simulink model "decoderapp"  (R2017b)
settings: Solver=FixedStepAuto  StartTime=0.0  StopTime=inf  RelTol=1e-3
libraries: androidlib x10, dspstat3 x2
settings Model: Creator=eslac_000  LastModifiedBy=eslac_000
settings OptimizationCC: PassReuseOutputArgsAs=Individual arguments  MaxStackSize=64
settings DebuggingCC: ParameterTunabilityLossMsg=error
settings HardwareCC: ProdBitPerPointer=32  ProdBitPerSizeT=32  ProdBitPerPtrDiffT=32  ProdLargestAtomicInteger=Long  ProdLargestAtomicFloat=Double  ProdWordSize=32  ProdHWDeviceType=ARM Compatible->ARM Cortex
settings SFSimCC: MATLABDynamicMemAlloc=off
settings RTWCC: SystemTargetFile=ert.tlc  HardwareBoard=Android Device  TemplateMakefile=ert_default_tmf  GenerateReport=on  Toolchain=Android SDK/NDK Tools  IncludeHyperlinkInReport=on  LaunchReport=on  GenerateTraceInfo=on  GenerateTraceReport=on  GenerateTraceReportSl=on  GenerateTraceReportSf=on  GenerateTraceReportEml=on
settings CodeAppCC: ForceParamTrailComments=on  IgnoreCustomStorageClasses=off  OperatorAnnotations=on  SimulinkDataObjDesc=on  SFDataObjDesc=on  InsertBlockDesc=on
settings ERTTargetCC: SupportVariableSizeSignals=on

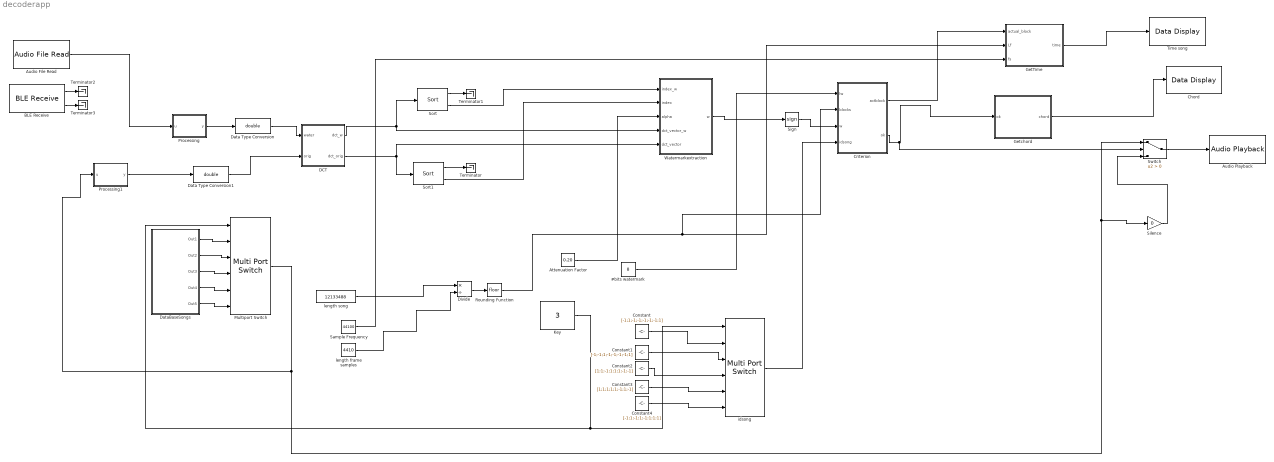
== system decoderapp ==
  " BLE Receive" : androidlib/ BLE Receive  DeviceMode=Central (Client)  device=No devices  character=No Characteristics  CustomService=off  ServiceName=Heart Rate  CharacteristicName="Heart Rate  Measurement"  CustomServiceUUID=<Enter Service UUID>  CustomCharUUID=<Enter Characteristic UUID>  DataSize=8  SampleTime=0.1  charseruuid=<empty>  seruuid=00001810-0000-1000-8000-00805f9b34fb  PeripheralService=0000180d-0000-1000-8000-00805f9b34fb  PeripheralCharacteristic=00002a37-0000-1000-8000-00805f9b34fb  chruuid=00002a37-0000-1000-8000-00805f9b34fb  BLEId=decoderapp/_BLE_Receive  IsCustomService=0
      settings: SourceProductName=Simulink Support Package for Android Devices  SourceProductBaseCode=ANDROID
  " length song" : Constant  Value=12133488
  "#bits watermark " : Constant  Value=8
  Attenuation Factor : Constant  Value=0.20
  Audio File Read : androidlib/Audio File Read  FileName=C:\Users\eslac_000\Desktop\UNIVERSIDAD\P2SEMESTRE\TESI\lab2_files\audio_watermarked.wav  FrameSize=4410
      settings: SourceProductName=Simulink Support Package for Android Devices  SourceProductBaseCode=ANDROID
  Audio Playback : androidlib/Audio Playback  SampleFreq=44100  AudioSamplingFreq=44100  SampleTime=0.1  DeviceStr=0  QueueDuration=0  BlockPlatform=Android
      settings: SourceProductName=Simulink Support Package for Android Devices  SourceProductBaseCode=ANDROID
  Chord : androidlib/Data Display  DataDisplayId=decoderapp/Chord  Format=Integer  Precision=6  SimulateUsing=Code generation  blockPlatform=Android
      settings: SourceProductName=Simulink Support Package for Android Devices  SourceProductBaseCode=ANDROID
  Constant : Constant  Value=[-1;1;-1;-1;-1;-1;-1;1]
  Constant1 : Constant  Value=[-1;-1;1;-1;-1;-1;-1;1]
  Constant2 : Constant  Value=[1;1;-1;1;1;1;-1;-1]
  Constant3 : Constant  Value=[1;1;1;1;1;-1;1;-1]
  Constant4 : Constant  Value=[-1;1;-1;1;-1;1;1;1]
  Criterion : MATLAB Function  TreatAsAtomicUnit=on
  "DCT " : MATLAB Function  TreatAsAtomicUnit=on
  Data Type Conversion : DataTypeConversion  OutDataTypeStr=double
  Data Type Conversion1 : DataTypeConversion  OutDataTypeStr=double
  DataBaseSongs : Subsystem
  Divide : Product  Inputs=*/
  GetTime : MATLAB Function  TreatAsAtomicUnit=on
  Getchord : MATLAB Function  TreatAsAtomicUnit=on
  "Key " : Constant  Value=3
  Multiport Switch : MultiPortSwitch  Inputs=5
  Processing : MATLAB Function  TreatAsAtomicUnit=on
  Processing1 : MATLAB Function  TreatAsAtomicUnit=on
  Rounding Function : Rounding
  Sample Frequency : Constant  Value=44100
  Sign : Signum
  Silence : Gain  Gain=0
  Sort : dspstat3/Sort  otype=Value and Index  dir=Descending  sortAlg=Quick sort  accumDataTypeStr=Inherit: Same as product output  accumLastDataTypeStr=Inherit: Same as product output  roundingMode=Floor  overflowMode=off
      settings: SourceProductName=DSP System Toolbox  SourceProductBaseCode=DS
  Sort1 : dspstat3/Sort  otype=Value and Index  dir=Descending  sortAlg=Quick sort  accumDataTypeStr=Inherit: Same as product output  accumLastDataTypeStr=Inherit: Same as product output  roundingMode=Floor  overflowMode=off
      settings: SourceProductName=DSP System Toolbox  SourceProductBaseCode=DS
  Switch : Switch  Criteria=u2 > Threshold
  Terminator{,1..3} (4 alike) : Terminator
  Time song : androidlib/Data Display  DataDisplayId=decoderapp/Time_song  Format=Float  Precision=6  SimulateUsing=Code generation  blockPlatform=Android
      settings: SourceProductName=Simulink Support Package for Android Devices  SourceProductBaseCode=ANDROID
  Watermarkextraction : MATLAB Function  TreatAsAtomicUnit=on
  idsong : MultiPortSwitch  Inputs=5
  length frame samples : Constant  Value=4410
  wires:
  "DCT "/1(dct_w) -> Sort/1, Watermarkextraction/4(dct_vector_w)
  "DCT "/2(dct_orig) -> Watermarkextraction/5(dct_vector), Sort1/1
  Multiport Switch/1 -> Silence/1, Switch/1, Processing1/1(u)
  Switch/1 -> Audio Playback/1
  DataBaseSongs/1(Out1) -> Multiport Switch/2
  DataBaseSongs/2(Out2) -> Multiport Switch/3
  DataBaseSongs/3(Out3) -> Multiport Switch/4
  DataBaseSongs/4(Out4) -> Multiport Switch/5
  Sort/2 -> Watermarkextraction/1(index_w)
  Sort1/2 -> Watermarkextraction/2(index)
  Sort1/1 -> Terminator/1
  Sort/1 -> Terminator1/1
  GetTime/1(time) -> Time song/1
  Getchord/1(chord) -> Chord/1
  Criterion/1(actblock) -> GetTime/1(actual_block)
  Criterion/2(ok) -> Switch/2, Getchord/1(ok)
  Data Type Conversion1/1 -> "DCT "/2(orig)
  Data Type Conversion/1 -> "DCT "/1(water)
  idsong/1 -> Criterion/4(idsong)
  Rounding Function/1 -> Criterion/2(blocks), GetTime/2(Lf)
  Sample Frequency/1 -> GetTime/3(fs)
  "#bits watermark "/1 -> Criterion/1(lw)
  Attenuation Factor/1 -> Watermarkextraction/3(alpha)
  " length song"/1 -> Divide/1
  Divide/1 -> Rounding Function/1
  length frame samples/1 -> Divide/2
  Constant3/1 -> idsong/5
  "Key "/1 -> idsong/1, Multiport Switch/1
  Constant2/1 -> idsong/4
  Constant1/1 -> idsong/3
  Constant/1 -> idsong/2
  Constant4/1 -> idsong/6
  Processing1/1(y) -> Data Type Conversion1/1
  Processing/1(y) -> Data Type Conversion/1
  Watermarkextraction/1(w) -> Sign/1
  Sign/1 -> Criterion/3(w)
  DataBaseSongs/5(Out5) -> Multiport Switch/6
  Audio File Read/1 -> Processing/1(u)
  Silence/1 -> Switch/3
  " BLE Receive"/1 -> Terminator2/1
  " BLE Receive"/2 -> Terminator3/1

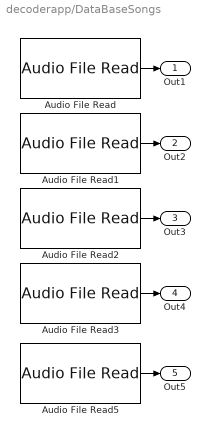
== system decoderapp/DataBaseSongs ==
  Audio File Read : androidlib/Audio File Read  FileName=C:\Users\eslac_000\Desktop\UNIVERSIDAD\P2SEMESTRE\TESI\lab2_files\songs\Musica ligera.mp3  FrameSize=4410
      settings: SourceProductName=Simulink Support Package for Android Devices  SourceProductBaseCode=ANDROID
  Audio File Read1 : androidlib/Audio File Read  FileName=C:\Users\eslac_000\Desktop\UNIVERSIDAD\P2SEMESTRE\TESI\lab2_files\songs\Nel blue.mp3  FrameSize=4410
      settings: SourceProductName=Simulink Support Package for Android Devices  SourceProductBaseCode=ANDROID
  Audio File Read2 : androidlib/Audio File Read  FileName=C:\Users\eslac_000\Desktop\UNIVERSIDAD\P2SEMESTRE\TESI\lab2_files\songs\howling.mp3  FrameSize=4410
      settings: SourceProductName=Simulink Support Package for Android Devices  SourceProductBaseCode=ANDROID
  Audio File Read3 : androidlib/Audio File Read  FileName=C:\Users\eslac_000\Desktop\UNIVERSIDAD\P2SEMESTRE\TESI\lab2_files\songs\rename.mp3  FrameSize=4410
      settings: SourceProductName=Simulink Support Package for Android Devices  SourceProductBaseCode=ANDROID
  Audio File Read5 : androidlib/Audio File Read  FileName=C:\Users\eslac_000\Desktop\UNIVERSIDAD\P2SEMESTRE\TESI\lab2_files\songs\vivalavida.mp3  FrameSize=4410
      settings: SourceProductName=Simulink Support Package for Android Devices  SourceProductBaseCode=ANDROID
  Out1 : Outport
  Out2 : Outport  Port=2
  Out3 : Outport  Port=3
  Out4 : Outport  Port=4
  Out5 : Outport  Port=5
  wires:
  Audio File Read2/1 -> Out3/1
  Audio File Read5/1 -> Out5/1
  Audio File Read3/1 -> Out4/1
  Audio File Read/1 -> Out1/1
  Audio File Read1/1 -> Out2/1

== matlab function decoderapp/GetTime ==
  data: actual_block input; Lf input; time output; fs input
function time  = fcn(actual_block,Lf,fs)
time=actual_block*Lf;%time in samples
time=time/fs;%time in seconds
% pause('on')
% pause(Lf/fs);
% pause('off');
end

== matlab function decoderapp/Watermarkextraction ==
  data: index_w input; index input; w output; alpha input; dct_vector_w input; dct_vector input
function w  = fcn(index_w,index,alpha,dct_vector_w,dct_vector)
    w=0;
    %str1 = sprintf('dct_vector_w(index(1, %d) = %s', i, dct_vector_w(index_w(1,i)));
    %disp(str1);
    %str2 = sprintf('dct_vector_n(index(1, %d) = %s', i, dct_vector(index(1,i)));
    %disp(str2);

    w= (dct_vector_w(index_w(1)) - dct_vector(index(1))) / alpha;
   
%     if isempty(w)
%         get=0;
%     else
%         get=1;
%     end
end

== matlab function decoderapp/Getchord ==
  data: ok input; chord output
function chord  = fcn(ok)
%prototype give a random chord
chord=uint8('.');
if(ok)
chords=['C' 'D' 'E' 'F' 'G' 'A' 'B'];
 chord = uint8( chords(randi(length(chords))));
end
end

== matlab function decoderapp/Criterion ==
  data: lw input; actblock output; blocks input; ok output; w input; idsong input
function [actblock,ok] = fcn(lw,blocks,w,idsong)
persistent M
persistent warn
persistent get
persistent idx
actblock=0;
ok=0;
 if isempty(M)
        M=0;
 end
     if isempty(warn)
        warn=0;
     end
     if isempty(get)
        get=0;
     end
     if isempty(idx)
        idx=0;
    end
if (~isempty(w))
    get=1;
end

while(get)
    M=M+1;
    idx=idx+1;
     if(M>blocks)
         get=0;
         break;
    end
    if(idx>lw)
        idx=1;
    end
    if(w~=idsong(idx))
        warn=warn+1;
    end
    if(warn<blocks/2)
        ok=1;
         actblock=M;
    else
        ok=0;
         actblock=M;
    end
    
   
   
end

== matlab function decoderapp/DCT  ==
  data: dct_w output; water input; orig input; dct_orig output
function [dct_w,dct_orig] = fcn(water,orig)
dct_w=zeros(length(water),1);
dct_orig=zeros(length(orig),1);
dct_orig=dct(orig,8192);
dct_w=dct(water,8192);
dct_orig=dct_orig(1:4410);
dct_w=dct_w(1:4410);
end

== matlab function decoderapp/Processing ==
  data: u input; y output
function y = fcn(u)
u=mean(u,2);
u=u-mean(u);
y = u;

== matlab function decoderapp/Processing1 ==
  data: u input; y output
function y = fcn(u)
u=mean(u,2);
u=u-mean(u);
y = u;
